simulink library "tgt"  (Simulink 8.1)
settings: Solver=ode1  StartTime=0.0  StopTime=Inf  FixedStep=0.001  RelTol=1e-3
PostLoadFcn:
  | , if any(exist('dsrtsu_mdlpostloadfcn', 'file') == [2, 3, 6]), try dsrtsu_mdlpostloadfcn('Execute', bdroot); catch fprintf('Error in PostLoadFcn (dsrtsu_mdlpostloadfcn) for model "%s":\n %s\n', bdroot, lasterr); end, end,
undefined symbols (not defined in the file or in its folder): KACC_TransitoryRelSpd_kph, KACC_TransitorySetTGapApproach_s, KACC_TransitorySetTGapIntrusion_s, KACC_TransitoryTGapDec_s
libraries: simulink x1, hcu_lib x1
settings Model: DSRTSU_INTERNAL_RTI_VER=450  DSRTSU_INTERNAL_RTI_TYPE=rti1401  RTICANMMDATA=struct('GeneralSetupData',struct('modelroot','D:\Projects\ELN150201\Repositories\Taiwan\trunk\AdasDragon\software\sw_development\arch\app\acc','generalsettings',struct('filesettings',struct('destfolder',struct('Name','RTICANMM_FILES','Check',1),'buildfolder',struct('Name','.','Check',1),'AbsDestfolder',struct('Name','D:\Projects\ELN150201\Repositories\Taiwan\trunk\AdasDragon\software\sw_development\arch\app\acc\RTICANMM_FILES'),'AbsBuildfolder',struct('Name','D:\Projects\ELN150201\Repositories\Taiwan\trunk\AdasDragon\software\sw_development\arch\app\acc'))),'options',struct('addpaths',1,'rmpaths',1,'addtrcexclusion',logical(1),'cannavigator',struct('checkmonitoring',0),'show_usrtrc',0,'use_usrtrc',0),'advanced',struct('options',[1 1 1 1 1 1 1 1 1 1 1 1 1 1 1 1 1 1 1 1 1 1 1 1 1 1 1 1 1 1 1 1 1 1 1 1 1 1 1 1 1 1 1 1 1 1 1 1 1 1 1 1 1 1 1 1 1 1 1 1 1 1 1 1 1 1 1 1 1 1 1 1 1 1 1 1 1 1 1 1 1 1 1 1 1 1 1 1 1 1 1 1 1 1 1 1 1 1 1 1]),'MPSetup',{{}},'modelname','Copy_of_scc','block','Copy_of_scc'))  DSRTSU_INTERNAL_RTIFPGA=40  Creator=AT015411  LastModifiedBy=AT015086

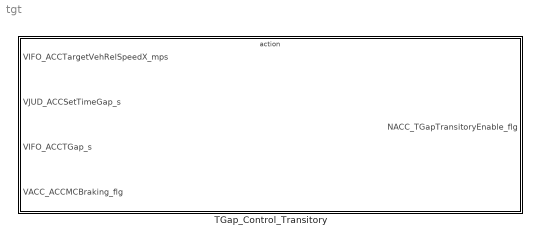
== system tgt ==
  TGap_Control_Transitory : Subsystem  TreatAsAtomicUnit=on

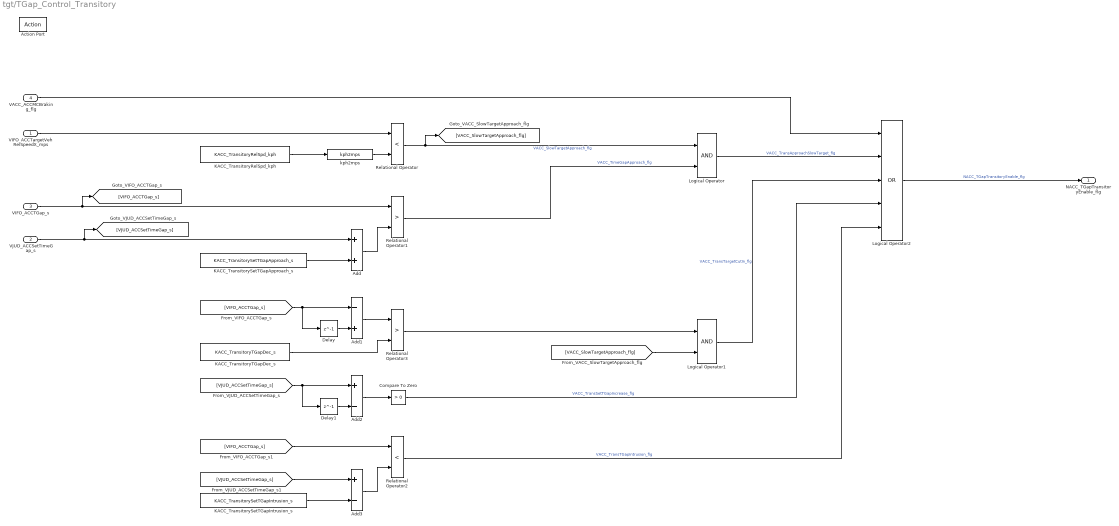
== system tgt/TGap_Control_Transitory ==
  VIFO_ACCTargetVehRelSpeedX_mps : Inport
  VJUD_ACCSetTimeGap_s : Inport  Port=2
  VIFO_ACCTGap_s : Inport  Port=3
  VACC_ACCMCBraking_flg : Inport  Port=4
  Action Port : ActionPort
  Add : Sum
  Add1 : Sum  Inputs=-+
  Add2 : Sum  Inputs=+-
  Add3 : Sum  Inputs=+-
  Compare To Zero : simulink/Logic and Bit Operations/Compare To Zero  relop=>  OutDataTypeStr=boolean
  Delay : Delay  DelayLength=1  InitialCondition=0
  Delay1 : Delay  DelayLength=1  InitialCondition=0
  KACC_TransitoryRelSpd_kph : Constant  Value=KACC_TransitoryRelSpd_kph
  KACC_TransitorySetTGapApproach_s : Constant  Value=KACC_TransitorySetTGapApproach_s
  KACC_TransitorySetTGapIntrusion_s : Constant  Value=KACC_TransitorySetTGapIntrusion_s
  KACC_TransitoryTGapDec_s : Constant  Value=KACC_TransitoryTGapDec_s
  Logical Operator : Logic  AllPortsSameDT=off  OutDataTypeStr=boolean
  Logical Operator1 : Logic  AllPortsSameDT=off  OutDataTypeStr=boolean
  Logical Operator2 : Logic  Operator=OR  Inputs=5  AllPortsSameDT=off  OutDataTypeStr=boolean
  Relational Operator : RelationalOperator  Operator=<  OutDataTypeStr=boolean
  Relational Operator1 : RelationalOperator  Operator=>  OutDataTypeStr=boolean
  Relational Operator2 : RelationalOperator  Operator=<  OutDataTypeStr=boolean
  Relational Operator3 : RelationalOperator  Operator=>  OutDataTypeStr=boolean
  kph2mps : hcu_lib/kph2mps
  NACC_TGapTransitoryEnable_flg : Outport
  wires:
  VIFO_ACCTargetVehRelSpeedX_mps/1 -> Relational Operator/1
  KACC_TransitoryRelSpd_kph/1 -> kph2mps/1
  kph2mps/1 -> Relational Operator/2
  VIFO_ACCTGap_s/1 -> [VIFO_ACCTGap_s], Relational Operator1/1
  VJUD_ACCSetTimeGap_s/1 -> [VJUD_ACCSetTimeGap_s], Add/1
  KACC_TransitorySetTGapApproach_s/1 -> Add/2
  Add/1 -> Relational Operator1/2
  Relational Operator/1 -> Logical Operator/1, [VACC_SlowTargetApproach_flg]  "VACC_SlowTargetApproach_flg"
  Relational Operator1/1 -> Logical Operator/2  "VACC_TimeGapApproach_flg"
  [VIFO_ACCTGap_s] -> Delay/1, Add1/1
  Delay/1 -> Add1/2
  Add1/1 -> Relational Operator3/1
  Relational Operator3/1 -> Logical Operator1/1
  [VACC_SlowTargetApproach_flg] -> Logical Operator1/2
  [VJUD_ACCSetTimeGap_s] -> Add2/1, Delay1/1
  Delay1/1 -> Add2/2
  Add2/1 -> Compare To Zero/1
  Compare To Zero/1 -> Logical Operator2/4  "VACC_TransSetTGapIncrease_flg"
  [VIFO_ACCTGap_s] -> Relational Operator2/1
  [VJUD_ACCSetTimeGap_s] -> Add3/1
  KACC_TransitorySetTGapIntrusion_s/1 -> Add3/2
  Add3/1 -> Relational Operator2/2
  Logical Operator/1 -> Logical Operator2/2  "VACC_TransApproachSlowTarget_flg"
  VACC_ACCMCBraking_flg/1 -> Logical Operator2/1
  Logical Operator1/1 -> Logical Operator2/3  "VACC_TransTargetCutIn_flg"
  Relational Operator2/1 -> Logical Operator2/5  "VACC_TransTGapIntrusion_flg"
  Logical Operator2/1 -> NACC_TGapTransitoryEnable_flg/1  "NACC_TGapTransitoryEnable_flg"
  KACC_TransitoryTGapDec_s/1 -> Relational Operator3/2
